simulink subsystem "ElectricalSystem"  (R2024b)
settings: Solver=VariableStepAuto  StartTime=0.0  StopTime=10.0  RelTol=1e-3
undefined symbols (not defined in the file): PlntDCDCVoltInit
settings Model: ModifiedByFormat=The MathWorks, Inc.  Creator=The MathWorks, Inc.  LastModifiedBy=The MathWorks, Inc.
settings RTWCC: GPUComputeCapability=3.5

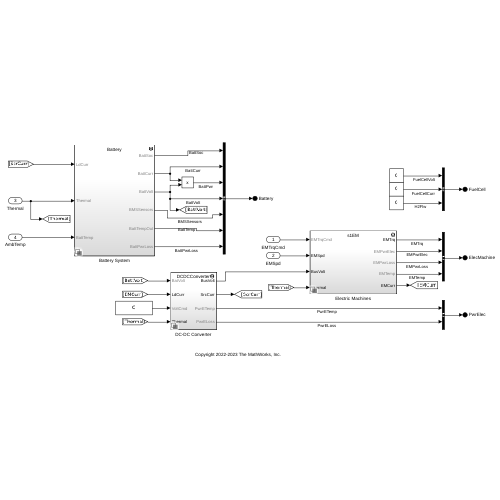
[thumbnail: Simulink's stored preview of the top-level diagram]
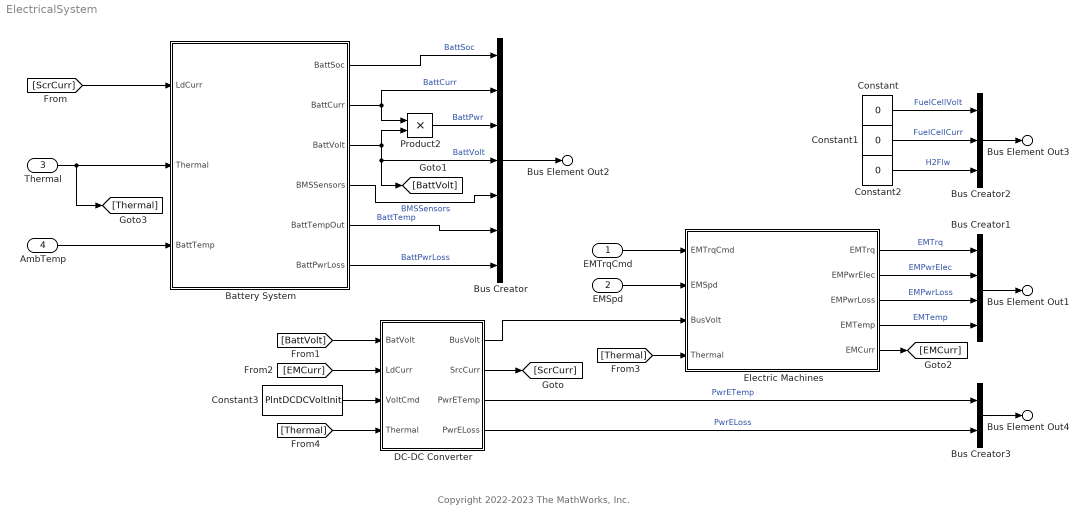
== system ElectricalSystem ==
  note: Copyright 2022-2023 The MathWorks, Inc.
  EMTrqCmd : Inport
  EMSpd : Inport  Port=2
  Thermal : Inport  Port=3
  AmbTemp : Inport  Port=4
  Battery System : Subsystem  Variant=on  VariantChoicesSpecifier={'Battery', 'IdealVoltageSource'}  VariantControlMode=label  LabelModeActiveChoice=Battery
  Bus Creator : BusCreator  Inputs=7
  Bus Creator1 : BusCreator  Inputs=4
  Bus Creator2 : BusCreator  Inputs=3
  Bus Creator3 : BusCreator  Inputs=2
  Constant : Constant  Value=0  SampleTime=-1
  Constant1 : Constant  Value=0  SampleTime=-1
  Constant2 : Constant  Value=0  SampleTime=-1
  Constant3 : Constant  Value=PlntDCDCVoltInit  SampleTime=-1
  DC-DC Converter : Subsystem  Variant=on  VariantChoicesSpecifier={'DCDCConverter', 'NoDCDCConverter'}  VariantControlMode=label  VariantControl=Choice  LabelModeActiveChoice=DCDCConverter
  Electric Machines : Subsystem  Variant=on  VariantChoicesSpecifier={'s1EM', 's2EM', 's3EM', 's4EM'}  VariantControlMode=label  LabelModeActiveChoice=s1EM
  Product2 : Product
  Bus Element Out2 : Outport  PortName=Battery
  Bus Element Out1 : Outport  Port=2  PortName=ElecMachine
  Bus Element Out3 : Outport  Port=3  PortName=FuelCell
  Bus Element Out4 : Outport  Port=4  PortName=PwrElec
  wires:
  Product2/1 -> Bus Creator/3  "BattPwr"
  Bus Creator2/1 -> Bus Element Out3/1
  Bus Creator1/1 -> Bus Element Out1/1
  Constant/1 -> Bus Creator2/1  "FuelCellVolt"
  Constant1/1 -> Bus Creator2/2  "FuelCellCurr"
  Bus Creator/1 -> Bus Element Out2/1
  Constant2/1 -> Bus Creator2/3  "H2Flw"
  Constant3/1 -> DC-DC Converter/3(VoltCmd)
  DC-DC Converter/2(SrcCurr) -> [ScrCurr]
  [BattVolt] -> DC-DC Converter/1(BatVolt)
  Bus Creator3/1 -> Bus Element Out4/1
  [EMCurr] -> DC-DC Converter/2(LdCurr)
  [ScrCurr] -> Battery System/1(LdCurr)
  Thermal/1 -> [Thermal], Battery System/2(Thermal)
  AmbTemp/1 -> Battery System/3(BattTemp)
  Battery System/1(BattSoc) -> Bus Creator/1  "BattSoc"
  Battery System/2(BattCurr) -> Product2/1, Bus Creator/2  "BattCurr"
  Battery System/6(BattPwrLoss) -> Bus Creator/7  "BattPwrLoss"
  Battery System/5(BattTempOut) -> Bus Creator/6  "BattTemp"
  Battery System/4(BMSSensors) -> Bus Creator/5  "BMSSensors"
  Battery System/3(BattVolt) -> [BattVolt], Bus Creator/4, Product2/2  "BattVolt"
  EMTrqCmd/1 -> Electric Machines/1(EMTrqCmd)
  EMSpd/1 -> Electric Machines/2(EMSpd)
  DC-DC Converter/1(BusVolt) -> Electric Machines/3(BusVolt)
  Electric Machines/1(EMTrq) -> Bus Creator1/1  "EMTrq"
  Electric Machines/2(EMPwrElec) -> Bus Creator1/2  "EMPwrElec"
  Electric Machines/5(EMCurr) -> [EMCurr]
  [Thermal] -> Electric Machines/4(Thermal)
  Electric Machines/3(EMPwrLoss) -> Bus Creator1/3  "EMPwrLoss"
  Electric Machines/4(EMTemp) -> Bus Creator1/4  "EMTemp"
  DC-DC Converter/3(PwrETemp) -> Bus Creator3/1  "PwrETemp"
  DC-DC Converter/4(PwrELoss) -> Bus Creator3/2  "PwrELoss"
  [Thermal] -> DC-DC Converter/4(Thermal)

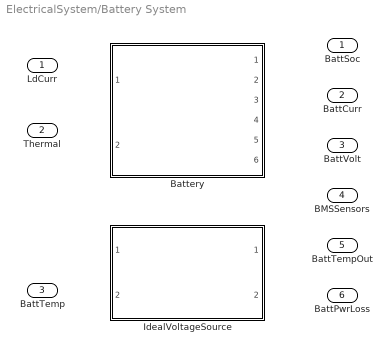
== system ElectricalSystem/Battery System ==
  LdCurr : Inport
  Thermal : Inport  Port=2
  BattTemp : Inport  Port=3
  Battery : Subsystem  VariantControl=Battery  ReferencedSubsystem=Battery
  IdealVoltageSource : Subsystem  VariantControl=IdealVoltageSource  ReferencedSubsystem=IdealVoltageSource
  BattSoc : Outport  VectorParamsAs1DForOutWhenUnconnected=off
  BattCurr : Outport  Port=2  VectorParamsAs1DForOutWhenUnconnected=off
  BattVolt : Outport  Port=3  VectorParamsAs1DForOutWhenUnconnected=off
  BMSSensors : Outport  Port=4  VectorParamsAs1DForOutWhenUnconnected=off
  BattTempOut : Outport  Port=5
  BattPwrLoss : Outport  Port=6

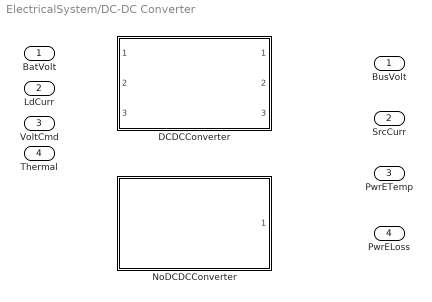
== system ElectricalSystem/DC-DC Converter ==
  BatVolt : Inport
  LdCurr : Inport  Port=2
  VoltCmd : Inport  Port=3
  Thermal : Inport  Port=4
  DCDCConverter : Subsystem  VariantControl=DCDCConverter  ReferencedSubsystem=DCDCConverter
  NoDCDCConverter : Subsystem  VariantControl=NoDCDCConverter  ReferencedSubsystem=NoDCDCConverter
  BusVolt : Outport
  SrcCurr : Outport  Port=2
  PwrETemp : Outport  Port=3
  PwrELoss : Outport  Port=4

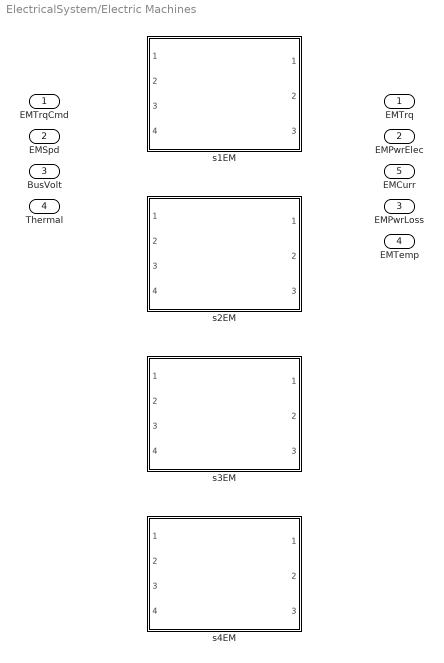
== system ElectricalSystem/Electric Machines ==
  EMTrqCmd : Inport
  EMSpd : Inport  Port=2
  BusVolt : Inport  Port=3
  Thermal : Inport  Port=4
  s1EM : Subsystem  VariantControl=s1EM  ReferencedSubsystem=s1EM
  s2EM : Subsystem  VariantControl=s2EM  ReferencedSubsystem=s2EM
  s3EM : Subsystem  VariantControl=s3EM  ReferencedSubsystem=s3EM
  s4EM : Subsystem  VariantControl=s4EM  ReferencedSubsystem=s4EM
  EMTrq : Outport
  EMPwrElec : Outport  Port=2
  EMPwrLoss : Outport  Port=3
  EMTemp : Outport  Port=4
  EMCurr : Outport  Port=5
